simulink model "gps_model"  (R2016b)
settings: Solver=VariableStepAuto  StartTime=0.0  StopTime=6000  RelTol=1e-3
undefined symbols (not defined in the file): fsw_params
libraries: gps x1, GPS_processing_lib x1, tle2eci_coarse_lib x1
settings Model: Creator=Taylor  LastModifiedBy=Taylor

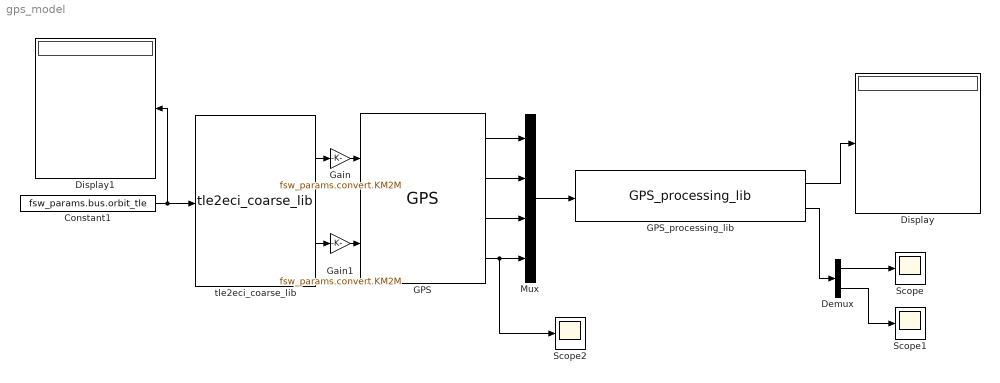
== system gps_model ==
  Constant1 : Constant  Value=fsw_params.bus.orbit_tle
  Demux : Demux  Outputs=2
  Display : Display
  Display1 : Display
  GPS : gps/GPS
  GPS_processing_lib : GPS_processing_lib/GPS_processing_lib
  Gain : Gain  Gain=fsw_params.convert.KM2M
  Gain1 : Gain  Gain=fsw_params.convert.KM2M
  Mux : Mux  Inputs=[3 3 2 1]
  Scope : Scope
  Scope1 : Scope
  Scope2 : Scope
  tle2eci_coarse_lib : tle2eci_coarse_lib/tle2eci_coarse_lib
  wires:
  GPS/1 -> Mux/1
  GPS/2 -> Mux/2
  GPS/4 -> Scope2/1, Mux/4
  Mux/1 -> GPS_processing_lib/1
  Constant1/1 -> Display1/1, tle2eci_coarse_lib/1
  tle2eci_coarse_lib/1 -> Gain/1
  GPS_processing_lib/1 -> Display/1
  GPS_processing_lib/2 -> Demux/1
  Demux/1 -> Scope/1
  Demux/2 -> Scope1/1
  GPS/3 -> Mux/3
  Gain/1 -> GPS/1
  tle2eci_coarse_lib/2 -> Gain1/1
  Gain1/1 -> GPS/2
